simulink model "Iris_DeePC_Control_Gazebo_Linear"  (R2022a)
settings: Solver=VariableStepAuto  StartTime=0.0  StopTime=sim_time  RelTol=1e-3
values from neighbouring files (symbols this model uses):
  accel_g = param.g    [DeePC_main.m]
  Ad = param.Ad_sys    [DeePC_main.m]    (also in collect_DeePC_data.m)
  Bd = param.Bd_sys    [DeePC_main.m]    (also in collect_DeePC_data.m)
  DeePC_param = evalin('base', 'DeePC_param')    [DeePC_Optimizer_osqp.m]
  K_pitch = param.K_lqr_outer_loop(3,8)    [DeePC_main.m]
  K_roll = param.K_lqr_outer_loop(2,7)    [DeePC_main.m]
  K_yaw = param.K_lqr_outer_loop(4,9)    [DeePC_main.m]
  Ki_xy = 0    [DeePC_main.m]
  Ki_z = 0    [DeePC_main.m]
  Kp_xy = - param.K_lqr_outer_loop(3,1)/param.K_lqr_outer_loop(2,7)    [DeePC_main.m]
  Kp_z = - param.K_lqr_outer_loop(1,3)    [DeePC_main.m]
  Kv_xy = - param.K_lqr_outer_loop(3,4)/param.K_lqr_outer_loop(2,7)    [DeePC_main.m]
  Kv_z = - param.K_lqr_outer_loop(1,6)    [DeePC_main.m]
  mass = param.nrotor_vehicle_mass_for_controller    [DeePC_main.m]
  param = evalin('base', 'param')    [DeePC_Optimizer_osqp.m]    (also in DeePC_main.m = load_crazyflie_parameters(); DeePC_update_uini_yini.m)
  start_time = 2    [DeePC_main.m]
undefined symbols (not defined in the file or in its folder): DiscIntNeverNeededParam
libraries: Crazyflie_Library x2
settings Model: Creator=ezzat  LastModifiedBy=simao
settings SolverCC: AlgebraicLoopSolver=LineSearch
settings DataIOCC: ReturnWorkspaceOutputs=off
settings DebuggingCC: UnconnectedInputMsg=warning  UnconnectedOutputMsg=warning  UnconnectedLineMsg=warning  SFMachineParentedDataDiag=warning  ArithmeticOperatorsInVariantConditions=warning
settings SFSimCC: CustomCodeUndefinedFunction=UseInterfaceOnly

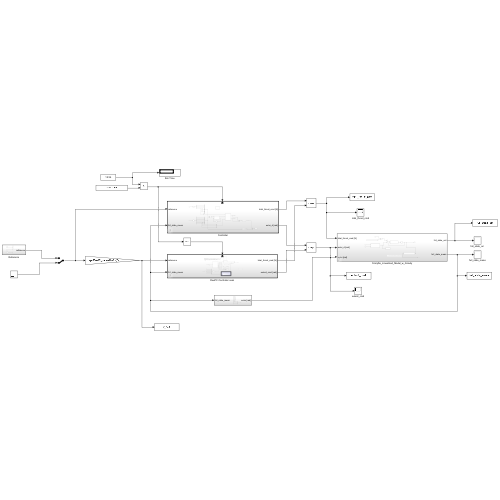
[thumbnail: Simulink's stored preview of the top-level diagram]
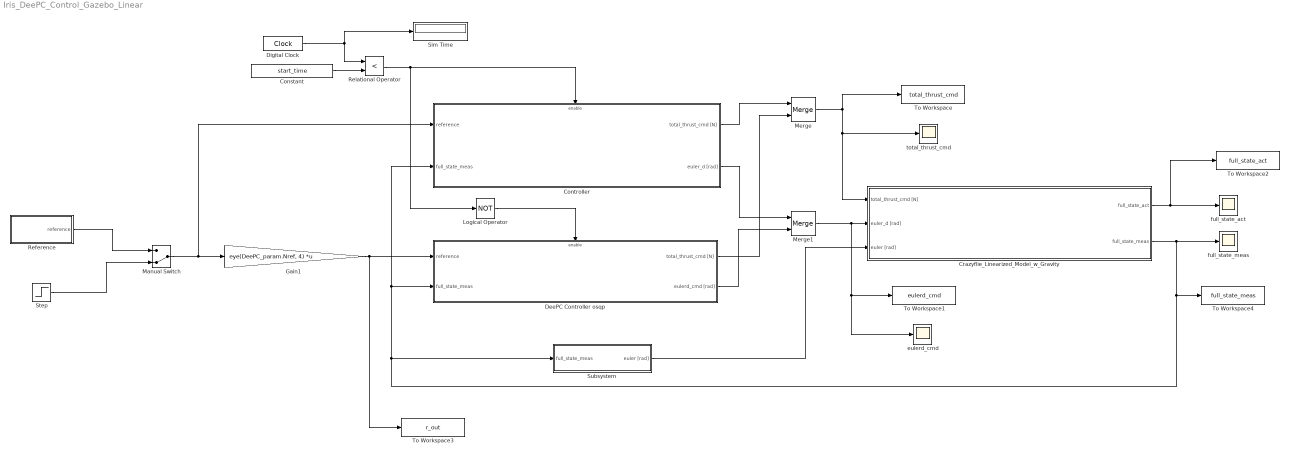
== system Iris_DeePC_Control_Gazebo_Linear ==
  Constant : Constant  Value=start_time
  Controller : Subsystem  AncestorBlock=Crazyflie_Library/LQR_Controller
  Crazyflie_Linearized_Model_w_Gravity : Subsystem  AncestorBlock=Crazyflie_Library/Crazyflie_Linearized_Model_w_Gravity
  DeePC Controller osqp : Subsystem  AncestorBlock=Crazyflie_Library/DeePC_Controller_osqp
  Digital Clock : DigitalClock  SampleTime=param.sample_time_controller_outer
  Gain1 : Gain  Gain=eye(DeePC_param.Nref, 4)  Multiplication=Matrix(K*u)
  Logical Operator : Logic  Operator=NOT  AllPortsSameDT=off  OutDataTypeStr=boolean
  Manual Switch : ManualSwitch  CurrentSetting=0
  Merge : Merge
  Merge1 : Merge
  Reference : Subsystem
  Relational Operator : RelationalOperator  Operator=<  OutDataTypeStr=boolean  RndMeth=Simplest  InputSameDT=off
  Sim Time : Display
  Step : Step  Time=start_time  Before=[param.nrotor_initial_condition(1:3); param.nrotor_initial_condition(9)]  After=[param.nrotor_final_condition(1:3); param.nrotor_final_condition(9)]  SampleTime=0
  Subsystem : Subsystem
  To Workspace : ToWorkspace  VariableName=total_thrust_cmd  SampleTime=param.sample_time_controller_outer
  To Workspace1 : ToWorkspace  VariableName=eulerd_cmd  SampleTime=param.sample_time_controller_outer
  To Workspace2 : ToWorkspace  VariableName=full_state_act  SampleTime=param.sample_time_controller_outer
  To Workspace3 : ToWorkspace  VariableName=r_out  SampleTime=param.sample_time_controller_outer
  To Workspace4 : ToWorkspace  VariableName=full_state_meas  SampleTime=param.sample_time_controller_outer
  eulerd_cmd : Scope
  full_state_act : Scope
  full_state_meas : Scope
  total_thrust_cmd : Scope
  wires:
  Crazyflie_Linearized_Model_w_Gravity/1(full_state_act) -> full_state_act/1, To Workspace2/1
  Crazyflie_Linearized_Model_w_Gravity/2(full_state_meas) -> Controller/2(full_state_meas), DeePC Controller osqp/2(full_state_meas), Subsystem/1(full_state_meas), To Workspace4/1, full_state_meas/1
  Digital Clock/1 -> Sim Time/1, Relational Operator/1
  Constant/1 -> Relational Operator/2
  DeePC Controller osqp/1(total_thrust_cmd [N]) -> Merge/2
  Merge/1 -> Crazyflie_Linearized_Model_w_Gravity/1(total_thrust_cmd [N]), total_thrust_cmd/1, To Workspace/1
  Merge1/1 -> Crazyflie_Linearized_Model_w_Gravity/2(euler_d [rad]), To Workspace1/1, eulerd_cmd/1
  DeePC Controller osqp/2(eulerd_cmd [rad]) -> Merge1/2
  Logical Operator/1 -> DeePC Controller osqp/Enable
  Gain1/1 -> DeePC Controller osqp/1(reference), To Workspace3/1
  Controller/1(total_thrust_cmd [N]) -> Merge/1
  Controller/2(euler_d [rad]) -> Merge1/1
  Subsystem/1(euler [rad]) -> Crazyflie_Linearized_Model_w_Gravity/3(euler [rad])
  Relational Operator/1 -> Controller/Enable, Logical Operator/1
  Manual Switch/1 -> Controller/1(reference), Gain1/1
  Step/1 -> Manual Switch/2
  Reference/1(reference) -> Manual Switch/1

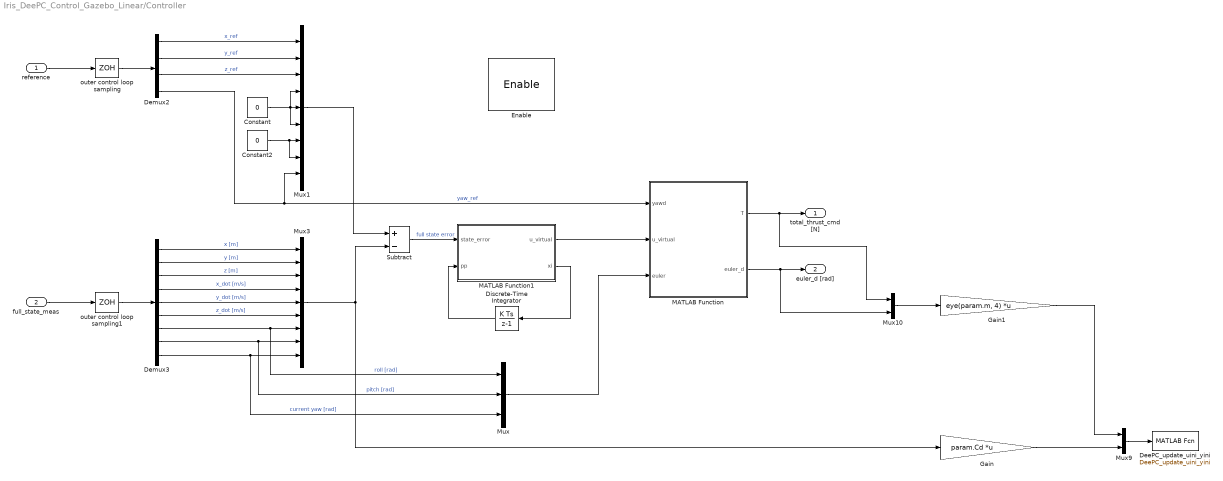
== system Iris_DeePC_Control_Gazebo_Linear/Controller ==
  reference : Inport
  full_state_meas : Inport  Port=2
  Enable : EnablePort
  Constant : Constant  Value=0
  Constant2 : Constant  Value=0
  DeePC_update_uini_yini : MATLABFcn  MATLABFcn=DeePC_update_uini_yini  OutputDimensions=0
  Demux2 : Demux
  Demux3 : Demux  Outputs=9
  Discrete-Time Integrator : DiscreteIntegrator  InitialCondition=[0;0;0]  SampleTime=-1  ICPrevOutput=DiscIntNeverNeededParam  ICPrevScaledInput=DiscIntNeverNeededParam
  Gain : Gain  Gain=param.Cd  Multiplication=Matrix(K*u)
  Gain1 : Gain  Gain=eye(param.m, 4)  Multiplication=Matrix(K*u)
  MATLAB Function : MATLAB Function  TreatAsAtomicUnit=on
  MATLAB Function1 : MATLAB Function  TreatAsAtomicUnit=on
  Mux : Mux  Inputs=3
  Mux1 : Mux  Inputs=9
  Mux10 : Mux  Inputs=2
  Mux3 : Mux  Inputs=9
  Mux9 : Mux  Inputs=2
  Subtract : Sum  Inputs=+-
  outer control loop sampling : ZeroOrderHold  SampleTime=param.sample_time_controller_outer
  outer control loop sampling1 : ZeroOrderHold  SampleTime=param.sample_time_controller_outer
  total_thrust_cmd [N] : Outport
  euler_d [rad] : Outport  Port=2
  wires:
  Mux3/1 -> Gain/1, Subtract/2
  Demux2/1 -> Mux1/1  "x_ref"
  Demux3/1 -> Mux3/1  "x [m]"
  Demux3/3 -> Mux3/3  "z [m]"
  Demux3/6 -> Mux3/6  "z_dot [m/s]"
  Constant/1 -> Mux1/5, Mux1/4, Mux1/6
  Constant2/1 -> Mux1/8, Mux1/7
  Demux3/2 -> Mux3/2  "y [m]"
  Demux2/4 -> Mux1/9, MATLAB Function/1(yawd)  "yaw_ref"
  Demux3/8 -> Mux/2, Mux3/8  "pitch [rad]"
  Demux3/9 -> Mux/3, Mux3/9  "current yaw [rad]"
  Demux3/7 -> Mux/1, Mux3/7  "roll [rad]"
  Demux2/2 -> Mux1/2  "y_ref"
  Demux3/4 -> Mux3/4  "x_dot [m/s]"
  Demux2/3 -> Mux1/3  "z_ref"
  Mux1/1 -> Subtract/1
  Demux3/5 -> Mux3/5  "y_dot [m/s]"
  full_state_meas/1 -> outer control loop sampling1/1
  outer control loop sampling/1 -> Demux2/1
  reference/1 -> outer control loop sampling/1
  outer control loop sampling1/1 -> Demux3/1
  Subtract/1 -> MATLAB Function1/1(state_error)  "full state error"
  Mux/1 -> MATLAB Function/3(euler)
  MATLAB Function1/2(xi) -> Discrete-Time Integrator/1
  Discrete-Time Integrator/1 -> MATLAB Function1/2(pp)
  MATLAB Function1/1(u_virtual) -> MATLAB Function/2(u_virtual)
  MATLAB Function/1(T) -> Mux10/1, total_thrust_cmd [N]/1
  MATLAB Function/2(euler_d) -> euler_d [rad]/1, Mux10/2
  Mux9/1 -> DeePC_update_uini_yini/1
  Mux10/1 -> Gain1/1
  Gain/1 -> Mux9/2
  Gain1/1 -> Mux9/1

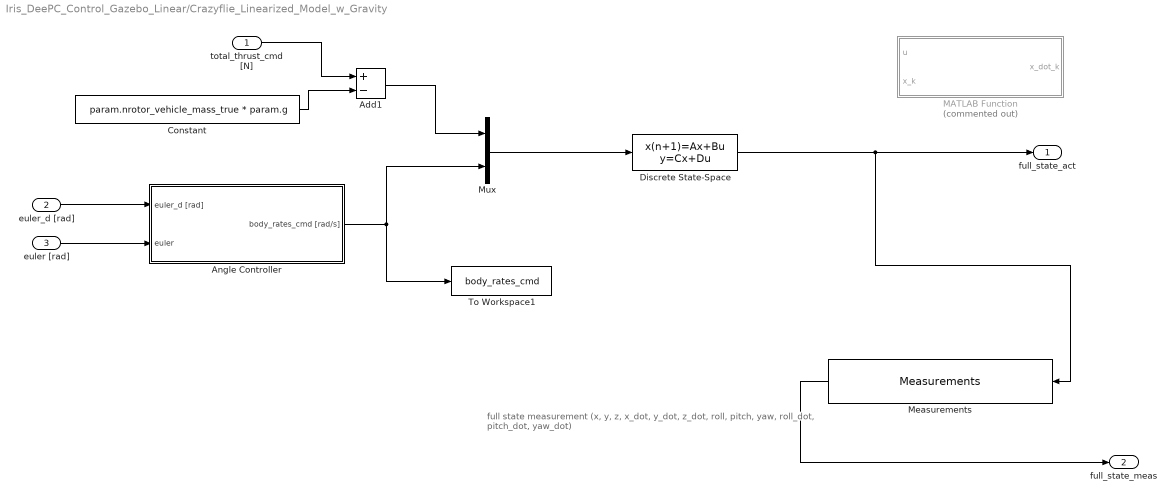
== system Iris_DeePC_Control_Gazebo_Linear/Crazyflie_Linearized_Model_w_Gravity ==
  note: full state measurement
      | (x, y, z, x_dot, y_dot, z_dot, roll, pitch, yaw, roll_dot, pitch_dot, yaw_dot)
  total_thrust_cmd [N] : Inport
  euler_d [rad] : Inport  Port=2
  euler [rad] : Inport  Port=3
  Add1 : Sum  Inputs=+-
  Angle Controller : Subsystem
  Constant : Constant  Value=param.nrotor_vehicle_mass_true * param.g
  Discrete State-Space : DiscreteStateSpace  A=param.Ad_sys  B=param.Bd_sys  C=eye(9)  D=zeros(9,4)  InitialCondition=param.nrotor_initial_condition(1:9)  SampleTime=0.04
  MATLAB Function : MATLAB Function  Commented=on  TreatAsAtomicUnit=on
  Measurements : Crazyflie_Library/Crazyflie_Linearized_Model_w_Gravity/Measurements  SystemSampleTime=-1  VariantActivationTime=update diagram  Latency=0  AutoFrameSizeCalculation=off
  Mux : Mux  Inputs=2
  To Workspace1 : ToWorkspace  VariableName=body_rates_cmd  SampleTime=param.sample_time_controller_outer
  full_state_act : Outport  VectorParamsAs1DForOutWhenUnconnected=off
  full_state_meas : Outport  Port=2  VectorParamsAs1DForOutWhenUnconnected=off
  wires:
  Discrete State-Space/1 -> Measurements/1, full_state_act/1
  total_thrust_cmd [N]/1 -> Add1/1
  Add1/1 -> Mux/1
  Constant/1 -> Add1/2
  Angle Controller/1(body_rates_cmd [rad/s]) -> To Workspace1/1, Mux/2
  euler_d [rad]/1 -> Angle Controller/1(euler_d [rad])
  euler [rad]/1 -> Angle Controller/2(euler)
  Measurements/1 -> full_state_meas/1
  Mux/1 -> Discrete State-Space/1

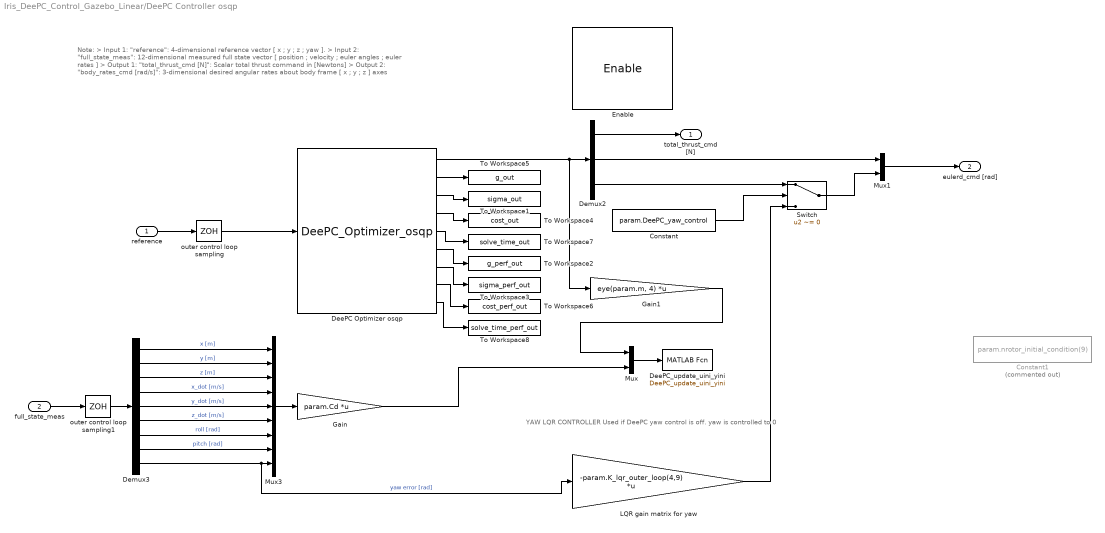
== system Iris_DeePC_Control_Gazebo_Linear/DeePC Controller osqp ==
  note: YAW LQR CONTROLLER
      | Used if DeePC yaw control is off. yaw is controlled to 0
  note: Note:
      | > Input 1: "reference": 4-dimensional reference vector [ x ; y ; z ; yaw ].
      | > Input 2: "full_state_meas": 12-dimensional measured full state vector [ position ; velocity ; euler angles ; euler rates ]
      | > Output 1: "total_thrust_cmd [N]": Scalar total thrust command in [Newtons]
      | > Output 2: "body_rates_cmd [rad/s]": 3-dimensional desired angular rates about body frame [ x ; y ; z ] axes
  reference : Inport
  full_state_meas : Inport  Port=2
  Enable : EnablePort
  Constant : Constant  Value=param.DeePC_yaw_control
  Constant1 : Constant  Commented=on  Value=param.nrotor_initial_condition(9)
  DeePC Optimizer osqp : Crazyflie_Library/DeePC_Optimizer_osqp  SystemSampleTime=-1  VariantActivationTime=update diagram  Latency=0  AutoFrameSizeCalculation=off
  DeePC_update_uini_yini : MATLABFcn  MATLABFcn=DeePC_update_uini_yini  OutputDimensions=0
  Demux2 : Demux  Outputs=[1 2 1]
  Demux3 : Demux  Outputs=9
  Gain : Gain  Gain=param.Cd  Multiplication=Matrix(K*u)
  Gain1 : Gain  Gain=eye(param.m, 4)  Multiplication=Matrix(K*u)
  LQR gain matrix for yaw : Gain  Gain=-param.K_lqr_outer_loop(4,9)  Multiplication=Matrix(K*u)
  Mux : Mux  Inputs=2
  Mux1 : Mux  Inputs=[2 1]
  Mux3 : Mux  Inputs=9
  Switch : Switch  Criteria=u2 ~= 0  SaturateOnIntegerOverflow=off  InputSameDT=off
  To Workspace1 : ToWorkspace  VariableName=sigma_out  SampleTime=-1
  To Workspace2 : ToWorkspace  VariableName=g_perf_out  SampleTime=-1
  To Workspace3 : ToWorkspace  VariableName=sigma_perf_out  SampleTime=-1
  To Workspace4 : ToWorkspace  VariableName=cost_out  SampleTime=-1
  To Workspace5 : ToWorkspace  VariableName=g_out  SampleTime=-1
  To Workspace6 : ToWorkspace  VariableName=cost_perf_out  SampleTime=-1
  To Workspace7 : ToWorkspace  VariableName=solve_time_out  SampleTime=-1
  To Workspace8 : ToWorkspace  VariableName=solve_time_perf_out  SampleTime=-1
  outer control loop sampling : ZeroOrderHold  SampleTime=param.sample_time_controller_outer
  outer control loop sampling1 : ZeroOrderHold  SampleTime=param.sample_time_controller_outer
  total_thrust_cmd [N] : Outport  VectorParamsAs1DForOutWhenUnconnected=off
  eulerd_cmd [rad] : Outport  Port=2  VectorParamsAs1DForOutWhenUnconnected=off
  wires:
  DeePC Optimizer osqp/7 -> To Workspace3/1
  DeePC Optimizer osqp/4 -> To Workspace4/1
  DeePC Optimizer osqp/3 -> To Workspace1/1
  DeePC Optimizer osqp/8 -> To Workspace6/1
  DeePC Optimizer osqp/6 -> To Workspace2/1
  DeePC Optimizer osqp/5 -> To Workspace7/1
  DeePC Optimizer osqp/9 -> To Workspace8/1
  DeePC Optimizer osqp/2 -> To Workspace5/1
  Gain1/1 -> Mux/1
  Constant/1 -> Switch/2
  Switch/1 -> Mux1/2
  Demux2/3 -> Switch/1
  Demux3/9 -> LQR gain matrix for yaw/1, Mux3/9  "yaw error [rad]"
  Mux1/1 -> eulerd_cmd [rad]/1
  Demux2/2 -> Mux1/1
  DeePC Optimizer osqp/1 -> Demux2/1, Gain1/1
  Gain/1 -> Mux/2
  Mux/1 -> DeePC_update_uini_yini/1
  outer control loop sampling/1 -> DeePC Optimizer osqp/1
  Demux2/1 -> total_thrust_cmd [N]/1
  Mux3/1 -> Gain/1
  outer control loop sampling1/1 -> Demux3/1
  reference/1 -> outer control loop sampling/1
  full_state_meas/1 -> outer control loop sampling1/1
  Demux3/5 -> Mux3/5  "y_dot [m/s]"
  Demux3/4 -> Mux3/4  "x_dot [m/s]"
  Demux3/7 -> Mux3/7  "roll [rad]"
  Demux3/8 -> Mux3/8  "pitch [rad]"
  Demux3/2 -> Mux3/2  "y [m]"
  Demux3/6 -> Mux3/6  "z_dot [m/s]"
  Demux3/3 -> Mux3/3  "z [m]"
  Demux3/1 -> Mux3/1  "x [m]"
  LQR gain matrix for yaw/1 -> Switch/3

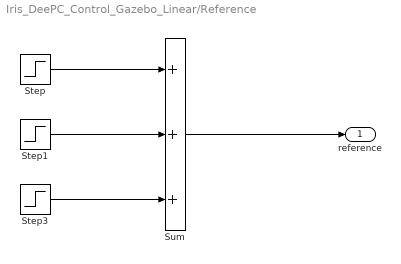
== system Iris_DeePC_Control_Gazebo_Linear/Reference ==
  Step : Step  Time=start_time  Before=[param.nrotor_initial_condition(1:3); param.nrotor_initial_condition(9)]  After=[param.nrotor_initial_condition(1:3) + 1; param.nrotor_initial_condition(9)]  SampleTime=0
  Step1 : Step  Time=start_time+20  Before=[0;0;0;0]  After=[-1;-1;-1;0]  SampleTime=0
  Step3 : Step  Time=start_time+40  Before=[0;0;0;0]  After=[1;1;1;0]  SampleTime=0
  Sum : Sum  Inputs=+++
  reference : Outport
  wires:
  Sum/1 -> reference/1
  Step/1 -> Sum/1
  Step1/1 -> Sum/2
  Step3/1 -> Sum/3

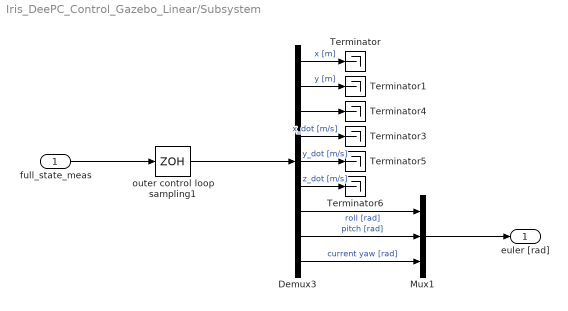
== system Iris_DeePC_Control_Gazebo_Linear/Subsystem ==
  full_state_meas : Inport
  Demux3 : Demux  Outputs=9
  Mux1 : Mux  Inputs=3
  Terminator{,1,3..6} (6 alike) : Terminator
  outer control loop sampling1 : ZeroOrderHold  SampleTime=param.sample_time_controller_outer
  euler [rad] : Outport
  wires:
  Demux3/7 -> Mux1/1  "roll [rad]"
  outer control loop sampling1/1 -> Demux3/1
  Demux3/8 -> Mux1/2  "pitch [rad]"
  full_state_meas/1 -> outer control loop sampling1/1
  Demux3/9 -> Mux1/3  "current yaw [rad]"
  Mux1/1 -> euler [rad]/1
  Demux3/1 -> Terminator/1  "x [m]"
  Demux3/2 -> Terminator1/1  "y [m]"
  Demux3/3 -> Terminator4/1
  Demux3/4 -> Terminator3/1  "x_dot [m/s]"
  Demux3/5 -> Terminator5/1  "y_dot [m/s]"
  Demux3/6 -> Terminator6/1  "z_dot [m/s]"

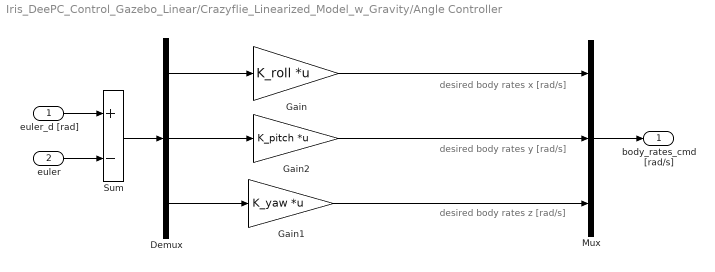
== system Iris_DeePC_Control_Gazebo_Linear/Crazyflie_Linearized_Model_w_Gravity/Angle Controller ==
  note: desired body rates x [rad/s]
  note: desired body rates z [rad/s]
  note: desired body rates y [rad/s]
  euler_d [rad] : Inport
  euler : Inport  Port=2
  Demux : Demux  Outputs=3
  Gain : Gain  Gain=K_roll  Multiplication=Matrix(K*u)
  Gain1 : Gain  Gain=K_yaw  Multiplication=Matrix(K*u)
  Gain2 : Gain  Gain=K_pitch  Multiplication=Matrix(K*u)
  Mux : Mux  Inputs=3
  Sum : Sum  Inputs=+-
  body_rates_cmd [rad/s] : Outport
  wires:
  euler_d [rad]/1 -> Sum/1
  euler/1 -> Sum/2
  Demux/2 -> Gain2/1
  Demux/3 -> Gain1/1
  Mux/1 -> body_rates_cmd [rad/s]/1
  Sum/1 -> Demux/1
  Gain2/1 -> Mux/2
  Gain1/1 -> Mux/3
  Gain/1 -> Mux/1
  Demux/1 -> Gain/1

== matlab function Iris_DeePC_Control_Gazebo_Linear/Crazyflie_Linearized_Model_w_Gravity/MATLAB Function ==
  data: u input; x_dot_k output; x_k input; Ad parameter; Bd parameter
function x_dot_k = fcn(u,x_k, Ad, Bd)

x_dot_k = zeros(9,1);

x_dot_k = Ad*x_k + Bd*u;

== matlab function Iris_DeePC_Control_Gazebo_Linear/Controller/MATLAB Function ==
  data: yawd input; u_virtual input; T output; euler_d output; euler input; mass parameter; accel_g parameter
function [T, euler_d] = input_transform(yawd, u_virtual, euler, mass, accel_g)

T = 0;
euler_d = zeros(3,1);

% Compute pitch, roll and T
Rz = eul2rotm([euler(3,1),0,0],'ZYX');

T_aux = mass * Rz'*(accel_g*[0;0;1] - u_virtual);
pitchd = atan2(T_aux(1),T_aux(3));
rolld = atan2(-T_aux(2),norm(T_aux([1,3])));
% pitchd = T_aux(1);
% rolld = -T_aux(2);

euler_d = [rolld;pitchd;yawd];

% T = norm(T_aux);
T = -u_virtual(3) + mass*accel_g;

== matlab function Iris_DeePC_Control_Gazebo_Linear/Controller/MATLAB Function1 ==
  data: state_error input; u_virtual output; pp input; xi output; Kp_xy parameter; Kv_xy parameter; Kv_z parameter; Ki_z parameter; Kp_z parameter; Ki_xy parameter
function [u_virtual,xi] = Controller(state_error, pp, Kp_xy, Kv_xy, Kv_z, Ki_z, Kp_z,Ki_xy)

p_err = state_error(1:3);
v_err = state_error(4:6);

u_virtual = zeros(3,1);
xi = zeros(3,1);

% Kv = -4;
% Kp = -4;
% Ki = 0;
% u = Kp*(p_err) + Kv*(v_err) + Ki*pp;
% u_virtual = u(:);

% Kp_xy = - 0.6552/3.6732;
% Kv_xy = - 0.7005/3.6732;
% 
% Kp_z = -0.3120;
% Kv_z = -0.9245;
% Ki = 0;

u_xy = Kv_xy*(v_err(1:2)) + Kp_xy*(p_err(1:2)) + Ki_xy*pp(1:2);

u_z = Kp_z*(p_err(3)) + Kv_z*(v_err(3)) + Ki_z*pp(3);

u_virtual = [u_xy;u_z];

xi = p_err;
